simulink model "ControllerDesign_Lat"  (R2017b)
settings: Solver=VariableStepAuto  StartTime=0.0  StopTime=5  RelTol=1e-3
undefined symbols (not defined in the file): Linmod
settings Model: Creator=One  LastModifiedBy=One

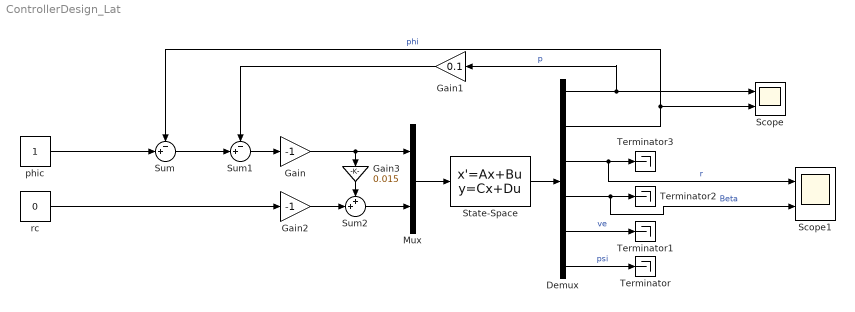
== system ControllerDesign_Lat ==
  Demux : Demux  Outputs=6
  Gain : Gain  Gain=-1
  Gain1 : Gain  Gain=0.1
  Gain2 : Gain  Gain=-1
  Gain3 : Gain  Gain=0.015
  Mux : Mux  Inputs=2
  Scope : Scope  NumInputPorts=2
  Scope1 : Scope  NumInputPorts=2
  State-Space : StateSpace  A=Linmod.Lat_5b.A  B=Linmod.Lat_5b.B  C=Linmod.Lat_5b.C  D=Linmod.Lat_5b.D  InitialCondition=0
  Sum : Sum  Inputs=-+|
  Sum1 : Sum  Inputs=-+|
  Sum2 : Sum  Inputs=++|
  Terminator{,1..3} (4 alike) : Terminator
  phic : Constant  SampleTime=0.01
  rc : Constant  Value=0  SampleTime=0.01
  wires:
  Mux/1 -> State-Space/1
  State-Space/1 -> Demux/1
  Demux/6 -> Terminator/1  "psi"
  Demux/5 -> Terminator1/1  "ve"
  Demux/4 -> Scope1/2, Terminator2/1  "Beta"
  Demux/2 -> Sum/1, Scope/2  "phi"
  Demux/1 -> Gain1/1, Scope/1  "p"
  Demux/3 -> Scope1/1, Terminator3/1  "r"
  phic/1 -> Sum/2
  Gain/1 -> Gain3/1, Mux/1
  Sum/1 -> Sum1/2
  Sum1/1 -> Gain/1
  Gain1/1 -> Sum1/1
  rc/1 -> Gain2/1
  Gain2/1 -> Sum2/2
  Sum2/1 -> Mux/2
  Gain3/1 -> Sum2/1
